simulink model "Lab1"  (R2018b)
settings: Solver=VariableStepAuto  StartTime=0.0  StopTime=0.02  RelTol=1e-3
settings Model: Creator=grecu  LastModifiedBy=grecu

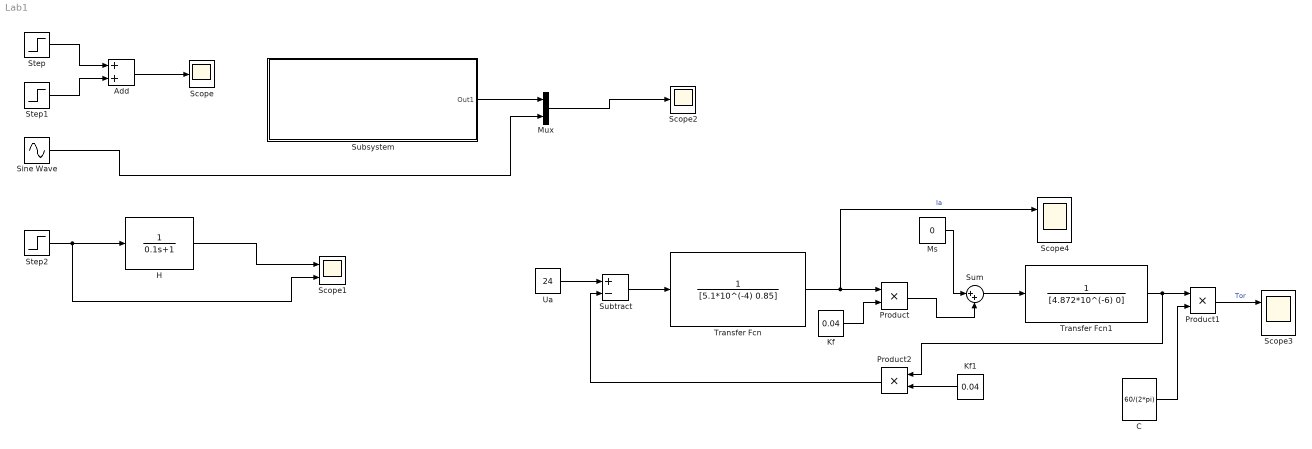
== system Lab1 ==
  Add : Sum
  C : Constant  Value=60/(2*pi)
  "H " : TransferFcn  Denominator=[0.1 1]
  Kf : Constant  Value=0.04
  Kf1 : Constant  Value=0.04
  Ms : Constant  Value=0
  Mux : Mux  Inputs=2
  Product : Product
  Product1 : Product
  Product2 : Product
  Scope : Scope
  Scope1 : Scope  NumInputPorts=2
  Scope2 : Scope
  Scope3 : Scope  NumInputPorts=2
  Scope4 : Scope  NumInputPorts=2
  Sine Wave : Sin  Amplitude=220*sqrt(2)  Frequency=60*2*pi  SampleTime=0
  Step : Step  Time=5  After=10  SampleTime=0
  Step1 : Step  Time=7  After=2  SampleTime=0
  Step2 : Step  After=0.5  SampleTime=0
  Subsystem : Subsystem
  Subtract : Sum  Inputs=+-
  Sum : Sum  Inputs=|++
  Transfer Fcn : TransferFcn  Denominator=[5.1*10^(-4) 0.85]
  Transfer Fcn1 : TransferFcn  Denominator=[4.872*10^(-6) 0]
  Ua : Constant  Value=24
  wires:
  Step/1 -> Add/1
  Add/1 -> Scope/1
  Step1/1 -> Add/2
  Sine Wave/1 -> Mux/2
  Subsystem/1(Out1) -> Mux/1
  Mux/1 -> Scope2/1
  "H "/1 -> Scope1/1
  Step2/1 -> Scope1/2, "H "/1
  Ua/1 -> Subtract/1
  Subtract/1 -> Transfer Fcn/1
  Transfer Fcn/1 -> Scope4/1, Product/1  "Ia"
  Kf/1 -> Product/2
  Ms/1 -> Sum/1
  Sum/1 -> Transfer Fcn1/1
  Transfer Fcn1/1 -> Product2/1, Product1/1
  Product1/1 -> Scope3/1  "Tor"
  C/1 -> Product1/2
  Product/1 -> Sum/2
  Kf1/1 -> Product2/2
  Product2/1 -> Subtract/2

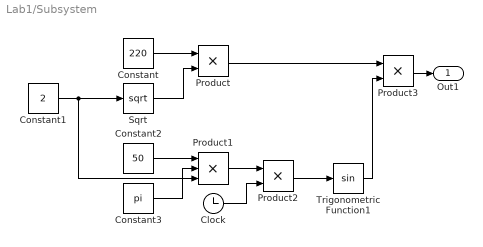
== system Lab1/Subsystem ==
  Clock : Clock
  Constant : Constant  Value=220
  Constant1 : Constant  Value=2
  Constant2 : Constant  Value=50
  Constant3 : Constant  Value=pi
  Product : Product
  Product1 : Product  Inputs=3
  Product2 : Product
  Product3 : Product
  Sqrt : Sqrt  SaturateOnIntegerOverflow=on
  Trigonometric Function1 : Trigonometry
  Out1 : Outport
  wires:
  Product3/1 -> Out1/1
  Product1/1 -> Product2/1
  Clock/1 -> Product2/2
  Constant1/1 -> Product1/3, Sqrt/1
  Constant/1 -> Product/1
  Constant3/1 -> Product1/2
  Trigonometric Function1/1 -> Product3/2
  Sqrt/1 -> Product/2
  Constant2/1 -> Product1/1
  Product/1 -> Product3/1
  Product2/1 -> Trigonometric Function1/1
